simulink subsystem "SerializeINT32"  (R2019b)
settings: Solver=VariableStepAuto  StartTime=0.0  StopTime=10.0  RelTol=1e-3
undefined symbols (not defined in the file or in its folder): __PRM__SERIALIZED__DATA__, SubsystemReferenceBlock
settings Model: Creator=VM  LastModifiedBy=VM

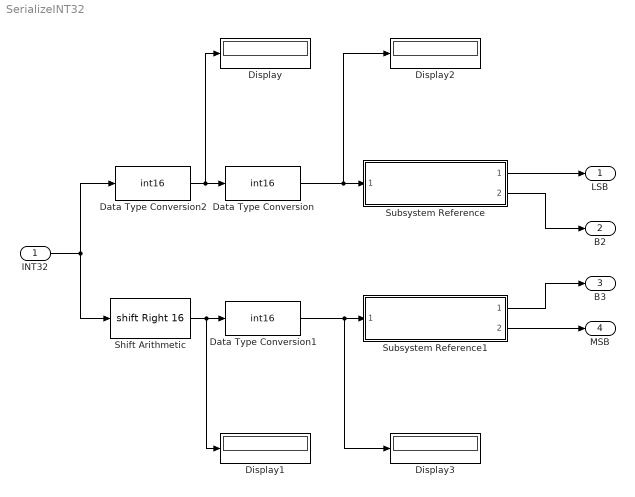
== system SerializeINT32 ==
  INT32 : Inport  OutDataTypeStr=int32
  Data Type Conversion : DataTypeConversion  OutDataTypeStr=int16
  Data Type Conversion1 : DataTypeConversion  OutDataTypeStr=int16
  Data Type Conversion2 : DataTypeConversion  OutDataTypeStr=int16  ConvertRealWorld=Stored Integer (SI)
  Display{,1..3} (4 alike) : Display
  Shift Arithmetic : ArithShift  BitShiftNumber=16  BitShiftDirection=Right
  Subsystem Reference : Subsystem  BlockKeywords=__PRM__SERIALIZED__DATA__:SubsystemReferenceBlock  ReferencedSubsystem=SerializeINT16
  Subsystem Reference1 : Subsystem  BlockKeywords=__PRM__SERIALIZED__DATA__:SubsystemReferenceBlock  ReferencedSubsystem=SerializeINT16
  LSB : Outport
  B2 : Outport  Port=2
  B3 : Outport  Port=3
  MSB : Outport  Port=4
  wires:
  Data Type Conversion1/1 -> Subsystem Reference1/1, Display3/1
  Shift Arithmetic/1 -> Data Type Conversion1/1, Display1/1
  Data Type Conversion/1 -> Display2/1, Subsystem Reference/1
  Subsystem Reference/1 -> LSB/1
  Subsystem Reference/2 -> B2/1
  Subsystem Reference1/1 -> B3/1
  Subsystem Reference1/2 -> MSB/1
  INT32/1 -> Data Type Conversion2/1, Shift Arithmetic/1
  Data Type Conversion2/1 -> Display/1, Data Type Conversion/1
